simulink model "simpleModel"  (R2016b)
settings: Solver=VariableStepAuto  StartTime=0.0  StopTime=10.0  RelTol=1e-3
model workspace (MAT data in the model file):
  K = 2
settings Model: Creator=Lenio  LastModifiedBy=Lenio

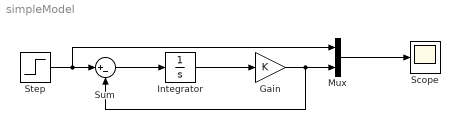
== system simpleModel ==
  Gain : Gain  Gain=K
  Integrator : Integrator
  Mux : Mux  Inputs=2
  Scope : Scope
  Step : Step  SampleTime=0
  Sum : Sum  Inputs=|+-
  wires:
  Step/1 -> Sum/1, Mux/1
  Sum/1 -> Integrator/1
  Integrator/1 -> Gain/1
  Gain/1 -> Sum/2, Mux/2
  Mux/1 -> Scope/1
